simulink model "battery_manager_Harness1"  (R2020b)
settings: Solver=FixedStepDiscrete  StartTime=0.0  StopTime=10.0  FixedStep=ContIntTime  RelTol=1e-3
settings Model: DataDictionary=battery_manager.sldd  Creator=RomanHaziev  LastModifiedBy=RomanHaziev

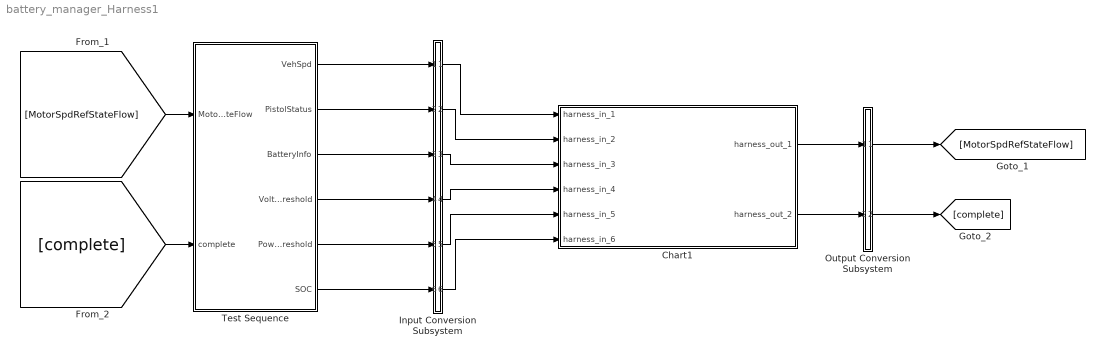
== system battery_manager_Harness1 ==
  Chart1 : Subsystem  Tag=__SL_testing_harness_stub_
  Input Conversion Subsystem : Subsystem  Tag=__SLT_ICS__  Description=|
      | Signal spec.
      | and routing
      settings: AttributesFormatString=%<Description>
  Output Conversion Subsystem : Subsystem  Tag=__SLT_OCS__  Description=|
      | Signal spec.
      | and routing
      settings: AttributesFormatString=%<Description>
  Test Sequence : Test Sequence  TreatAsAtomicUnit=on
  wires:
  Test Sequence/1(VehSpd) -> Input Conversion Subsystem/1(Inport_1)
  Test Sequence/2(PistolStatus) -> Input Conversion Subsystem/2(Inport_2)
  Test Sequence/3(BatteryInfo) -> Input Conversion Subsystem/3(Inport_3)
  Test Sequence/4(VoltageThreshold) -> Input Conversion Subsystem/4(Inport_4)
  Test Sequence/5(PowerThreshold) -> Input Conversion Subsystem/5(Inport_5)
  Test Sequence/6(SOC) -> Input Conversion Subsystem/6(Inport_6)
  [MotorSpdRefStateFlow] -> Test Sequence/1(MotorSpdRefStateFlow)
  [complete] -> Test Sequence/2(complete)
  Output Conversion Subsystem/1(Outport_1) -> [MotorSpdRefStateFlow]
  Output Conversion Subsystem/2(Outport_2) -> [complete]
  Input Conversion Subsystem/1(Outport_1) -> Chart1/1(harness_in_1)
  Input Conversion Subsystem/2(Outport_2) -> Chart1/2(harness_in_2)
  Input Conversion Subsystem/3(Outport_3) -> Chart1/3(harness_in_3)
  Input Conversion Subsystem/4(Outport_4) -> Chart1/4(harness_in_4)
  Input Conversion Subsystem/5(Outport_5) -> Chart1/5(harness_in_5)
  Input Conversion Subsystem/6(Outport_6) -> Chart1/6(harness_in_6)
  Chart1/1(harness_out_1) -> Output Conversion Subsystem/1(Inport_1)
  Chart1/2(harness_out_2) -> Output Conversion Subsystem/2(Inport_2)

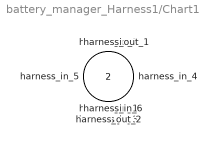
== system battery_manager_Harness1/Chart1 ==
  harness_in_1 : Inport
  harness_in_2 : Inport  Port=2
  harness_in_3 : Inport  Port=3
  harness_in_4 : Inport  Port=4
  harness_in_5 : Inport  Port=5
  harness_in_6 : Inport  Port=6
  harness_out_1 : Outport
  harness_out_2 : Outport  Port=2

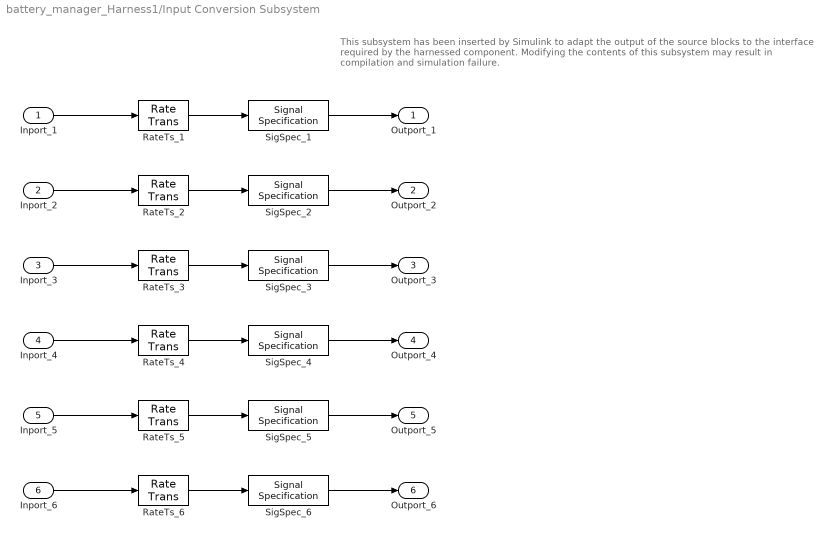
== system battery_manager_Harness1/Input Conversion Subsystem ==
  note: This subsystem has been inserted by Simulink to adapt the output of the source blocks to the interface required by the harnessed component.
      |  Modifying the contents of this subsystem may result in compilation and simulation failure.
  Inport_1 : Inport
  Inport_2 : Inport  Port=2
  Inport_3 : Inport  Port=3
  Inport_4 : Inport  Port=4
  Inport_5 : Inport  Port=5
  Inport_6 : Inport  Port=6
  RateTs_{1..2,4..6} (5 alike) : RateTransition  OutPortSampleTime=0.004
  RateTs_3 : RateTransition  OutPortSampleTime=[-1, 0]
  SigSpec_1 : SignalSpecification  OutDataTypeStr=single  Dimensions=[1]  SampleTime=0.004
  SigSpec_2 : SignalSpecification  OutDataTypeStr=Enum: EnumPistSt  Dimensions=[1]  SampleTime=0.004
  SigSpec_3 : SignalSpecification  OutDataTypeStr=double  Dimensions=[1]  SampleTime=[-1, 0]
  SigSpec_4 : SignalSpecification  OutDataTypeStr=boolean  Dimensions=[1]  SampleTime=0.004
  SigSpec_5 : SignalSpecification  OutDataTypeStr=boolean  Dimensions=[1]  SampleTime=0.004
  SigSpec_6 : SignalSpecification  OutDataTypeStr=single  Dimensions=[1]  SampleTime=0.004
  Outport_1 : Outport
  Outport_2 : Outport  Port=2
  Outport_3 : Outport  Port=3
  Outport_4 : Outport  Port=4
  Outport_5 : Outport  Port=5
  Outport_6 : Outport  Port=6
  wires:
  SigSpec_1/1 -> Outport_1/1
  RateTs_1/1 -> SigSpec_1/1
  Inport_1/1 -> RateTs_1/1
  SigSpec_2/1 -> Outport_2/1
  RateTs_2/1 -> SigSpec_2/1
  Inport_2/1 -> RateTs_2/1
  SigSpec_3/1 -> Outport_3/1
  RateTs_3/1 -> SigSpec_3/1
  Inport_3/1 -> RateTs_3/1
  SigSpec_4/1 -> Outport_4/1
  RateTs_4/1 -> SigSpec_4/1
  Inport_4/1 -> RateTs_4/1
  SigSpec_5/1 -> Outport_5/1
  RateTs_5/1 -> SigSpec_5/1
  Inport_5/1 -> RateTs_5/1
  SigSpec_6/1 -> Outport_6/1
  RateTs_6/1 -> SigSpec_6/1
  Inport_6/1 -> RateTs_6/1

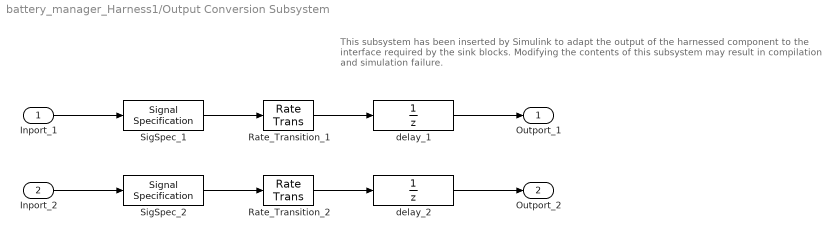
== system battery_manager_Harness1/Output Conversion Subsystem ==
  note: This subsystem has been inserted by Simulink to adapt the output of the harnessed component to the interface required by the sink blocks.
      |  Modifying the contents of this subsystem may result in compilation and simulation failure.
  Inport_1 : Inport
  Inport_2 : Inport  Port=2
  Rate_Transition_1 : RateTransition  OutPortSampleTimeOpt=Inherit
  Rate_Transition_2 : RateTransition  OutPortSampleTimeOpt=Inherit
  SigSpec_1 : SignalSpecification  OutDataTypeStr=double  Dimensions=[1]  SampleTime=0.004
  SigSpec_2 : SignalSpecification  OutDataTypeStr=double  Dimensions=[1]  SampleTime=0.004
  delay_1 : UnitDelay  SampleTime=-1
  delay_2 : UnitDelay  SampleTime=-1
  Outport_1 : Outport
  Outport_2 : Outport  Port=2
  wires:
  Inport_1/1 -> SigSpec_1/1
  SigSpec_1/1 -> Rate_Transition_1/1
  Rate_Transition_1/1 -> delay_1/1
  delay_1/1 -> Outport_1/1
  Inport_2/1 -> SigSpec_2/1
  SigSpec_2/1 -> Rate_Transition_2/1
  Rate_Transition_2/1 -> delay_2/1
  delay_2/1 -> Outport_2/1

== stateflow chart battery_manager_Harness1/Test Sequence ==
  settings: updateMethod=DISCRETE  sampleTime=0.004  stateMachineType=SIMPLIFIED_MACHINE
  state Run
    %% Initialize data outputs.
    VehSpd = single(0);
    PistolStatus = EnumPistSt.NA;
    BatteryInfo = 0;
    VoltageThreshold = false;
    PowerThreshold = false;
    SOC = single(0);
  (default) -> Run
  data: MotorSpdRefStateFlow input double size=[1]; complete input double size=[1]; VehSpd output single size=[1]; PistolStatus output Enum: EnumPistSt size=[1]; BatteryInfo output double size=[1]; VoltageThreshold output boolean size=[1]; PowerThreshold output boolean size=[1]; SOC output single size=[1]
